simulink model "SWC_VES_type"  (R2021b)
settings: Solver=FixedStepDiscrete  StartTime=0.0  StopTime=10.0  FixedStep=0.001  RelTol=1e-3
undefined symbols (not defined in the file or in its folder): R_HALINCDD_CSOP_IPCF_Handler
libraries: simulink x78
(part 1 of 2)
settings Model: DataDictionary=APPTypes.sldd  Creator=FVT23010  LastModifiedBy=FVT23033
settings DataIOCC: SaveFormat=StructureWithTime
settings OptimizationCC: DefaultParameterBehavior=Inlined  EnhancedBackFolding=on  PassReuseOutputArgsAs=Individual arguments  ZeroExternalMemoryAtStartup=off  ZeroInternalMemoryAtStartup=off  OptimizeBlockOrder=speed  DifferentSizesBufferReuse=on  OptimizationCustomize=off  EfficientTunableParamExpr=on
settings DebuggingCC: ParameterTunabilityLossMsg=error
settings HardwareCC: ProdBitPerPointer=32  ProdBitPerSizeT=32  ProdBitPerPtrDiffT=32  ProdLargestAtomicInteger=Long  ProdLargestAtomicFloat=Double  ProdWordSize=32  ProdLongLongMode=on  ProdHWDeviceType=ARM Compatible->ARM Cortex-M
settings ModelReferenceCC: ModelReferenceNumInstancesAllowed=Single
settings SFSimCC: MATLABDynamicMemAlloc=off
settings RTWCC: Description=AUTOSAR  SystemTargetFile=autosar.tlc  GenCodeOnly=on  TemplateMakefile=ert_default_tmf  PortableWordSizes=on
settings CodeAppCC: ForceParamTrailComments=on  IgnoreCustomStorageClasses=off  OperatorAnnotations=on  SimulinkDataObjDesc=on  SFDataObjDesc=on  InsertBlockDesc=on
settings STFCustomTargetCC: TargetLangStandard=C99 (ISO)  UtilityFuncGeneration=Shared location  MultiwordLength=256  ParMdlRefBuildCompliant=on  CompOptLevelCompliant=on  IncludeMdlTerminateFcn=off  CombineOutputUpdateFcns=on  SuppressErrorStatus=on  ERTCustomFileBanners=on  SupportNonFinite=off  SupportComplex=off  SupportContinuousTime=off  SupportNonInlinedSFcns=off  RemoveResetFunc=on  MATLABClassNameForMDSCustomization=Simulink.SoftwareTarget.ERTCustomization  AutosarCompliant=on  GRTInterface=off  UseToolchainInfoCompliant=on  GenerateSharedConstants=off  LookupTableObjectStructAxisOrder=2,1,3,4,...  LUTObjectStructOrderEvenSpacing=Size,Table,Breakpoints  SystemTargetFile=autosar.tlc
settings ERTTargetCC: TargetLangStandard=C99 (ISO)  UtilityFuncGeneration=Shared location  ConcurrentExecutionCompliant=off  IncludeMdlTerminateFcn=off  SuppressErrorStatus=on  SupportNonFinite=off  SupportComplex=off  ModelStepFunctionPrototypeControlCompliant=off  CPPClassGenCompliant=off  AutosarCompliant=on  GenerateSharedConstants=off  LookupTableObjectStructAxisOrder=2,1,3,4,...  LUTObjectStructOrderEvenSpacing=Size,Table,Breakpoints  GenerateASAP2=on  InlinedParameterPlacement=NonHierarchical  ERTCustomFileTemplate=example_file_process.tlc  ConvertIfToSwitch=off  SuppressUnreachableDefaultCases=off  BooleanTrueId=true_MatlabRTW  BooleanFalseId=false_MatlabRTW

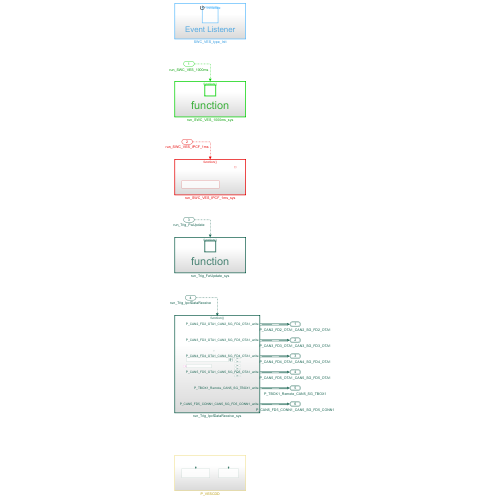
[thumbnail: Simulink's stored preview of the top-level diagram]
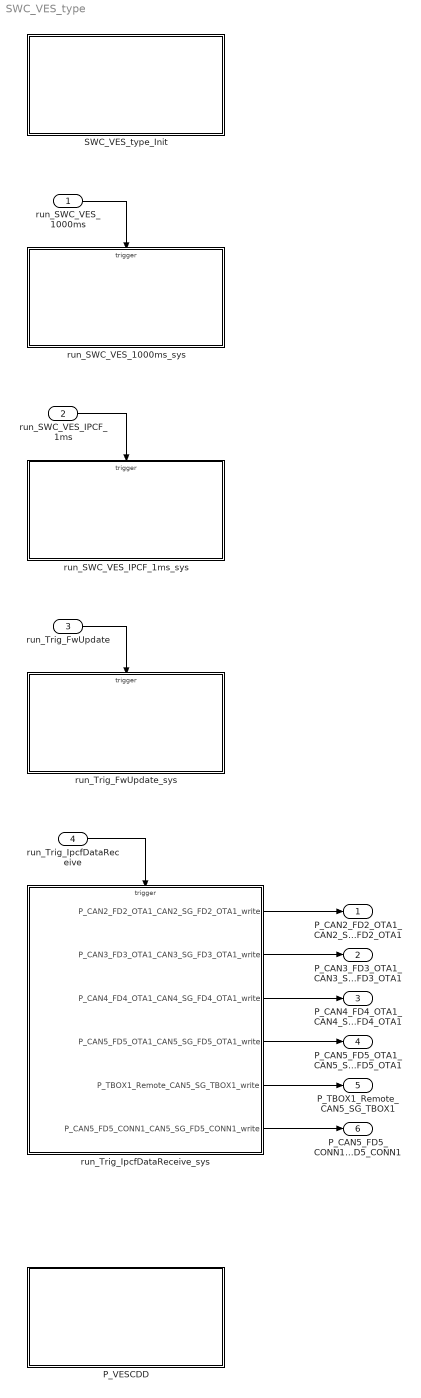
== system SWC_VES_type ==
  run_SWC_VES_1000ms : Inport  SampleTime=1  OutputFunctionCall=on
  run_SWC_VES_IPCF_1ms : Inport  Port=2  SampleTime=0.001  OutputFunctionCall=on
  run_Trig_FwUpdate : Inport  Port=3  OutputFunctionCall=on
  run_Trig_IpcfDataReceive : Inport  Port=4  OutputFunctionCall=on
  P_VESCDD : Subsystem
  SWC_VES_type_Init : Subsystem
  run_SWC_VES_1000ms_sys : Subsystem
  run_SWC_VES_IPCF_1ms_sys : Subsystem
  run_Trig_FwUpdate_sys : Subsystem
  run_Trig_IpcfDataReceive_sys : Subsystem
  P_CAN2_FD2_OTA1_CAN2_SG_FD2_OTA1 : Outport  OutDataTypeStr=Bus: DT_CAN2_SG_FD2_OTA1  PortDimensions=1  BusOutputAsStruct=on
  P_CAN3_FD3_OTA1_CAN3_SG_FD3_OTA1 : Outport  Port=2  OutDataTypeStr=Bus: DT_CAN3_SG_FD3_OTA1  PortDimensions=1  BusOutputAsStruct=on
  P_CAN4_FD4_OTA1_CAN4_SG_FD4_OTA1 : Outport  Port=3  OutDataTypeStr=Bus: DT_CAN4_SG_FD4_OTA1  PortDimensions=1  BusOutputAsStruct=on
  P_CAN5_FD5_OTA1_CAN5_SG_FD5_OTA1 : Outport  Port=4  OutDataTypeStr=Bus: DT_CAN5_SG_FD5_OTA1  PortDimensions=1  BusOutputAsStruct=on
  P_TBOX1_Remote_CAN5_SG_TBOX1 : Outport  Port=5  OutDataTypeStr=Bus: DT_CAN5_SG_TBOX1  PortDimensions=1  BusOutputAsStruct=on
  P_CAN5_FD5_CONN1_CAN5_SG_FD5_CONN1 : Outport  Port=6  OutDataTypeStr=Bus: DT_CAN5_SG_FD5_CONN1  PortDimensions=1  BusOutputAsStruct=on
  wires:
  run_Trig_IpcfDataReceive_sys/1(P_CAN2_FD2_OTA1_CAN2_SG_FD2_OTA1_write) -> P_CAN2_FD2_OTA1_CAN2_SG_FD2_OTA1/1
  run_Trig_IpcfDataReceive_sys/2(P_CAN3_FD3_OTA1_CAN3_SG_FD3_OTA1_write) -> P_CAN3_FD3_OTA1_CAN3_SG_FD3_OTA1/1
  run_Trig_IpcfDataReceive_sys/3(P_CAN4_FD4_OTA1_CAN4_SG_FD4_OTA1_write) -> P_CAN4_FD4_OTA1_CAN4_SG_FD4_OTA1/1
  run_Trig_IpcfDataReceive_sys/4(P_CAN5_FD5_OTA1_CAN5_SG_FD5_OTA1_write) -> P_CAN5_FD5_OTA1_CAN5_SG_FD5_OTA1/1
  run_Trig_IpcfDataReceive_sys/5(P_TBOX1_Remote_CAN5_SG_TBOX1_write) -> P_TBOX1_Remote_CAN5_SG_TBOX1/1
  run_Trig_IpcfDataReceive_sys/6(P_CAN5_FD5_CONN1_CAN5_SG_FD5_CONN1_write) -> P_CAN5_FD5_CONN1_CAN5_SG_FD5_CONN1/1
  run_SWC_VES_1000ms/1 -> run_SWC_VES_1000ms_sys/Trigger
  run_SWC_VES_IPCF_1ms/1 -> run_SWC_VES_IPCF_1ms_sys/Trigger
  run_Trig_FwUpdate/1 -> run_Trig_FwUpdate_sys/Trigger
  run_Trig_IpcfDataReceive/1 -> run_Trig_IpcfDataReceive_sys/Trigger

== system SWC_VES_type/P_VESCDD ==
  run_VESCDD_sys : Subsystem

== system SWC_VES_type/SWC_VES_type_Init ==
  Event Listener : EventListener  EventName=reset

== system SWC_VES_type/run_SWC_VES_1000ms_sys ==
  function : TriggerPort  TriggerType=function-call  VariantControl=(inherit)  SampleTimeType=periodic  SampleTime=-1

== system SWC_VES_type/run_SWC_VES_IPCF_1ms_sys ==
  function : TriggerPort  TriggerType=function-call  VariantControl=(inherit)  SampleTimeType=periodic  SampleTime=-1
  R_HALINCDD_CSOP_IPCF_Handler : FunctionCaller  FunctionPrototype=R_HALINCDD_CSOP_IPCF_Handler()

== system SWC_VES_type/run_Trig_FwUpdate_sys ==
  function : TriggerPort  TriggerType=function-call  VariantControl=(inherit)

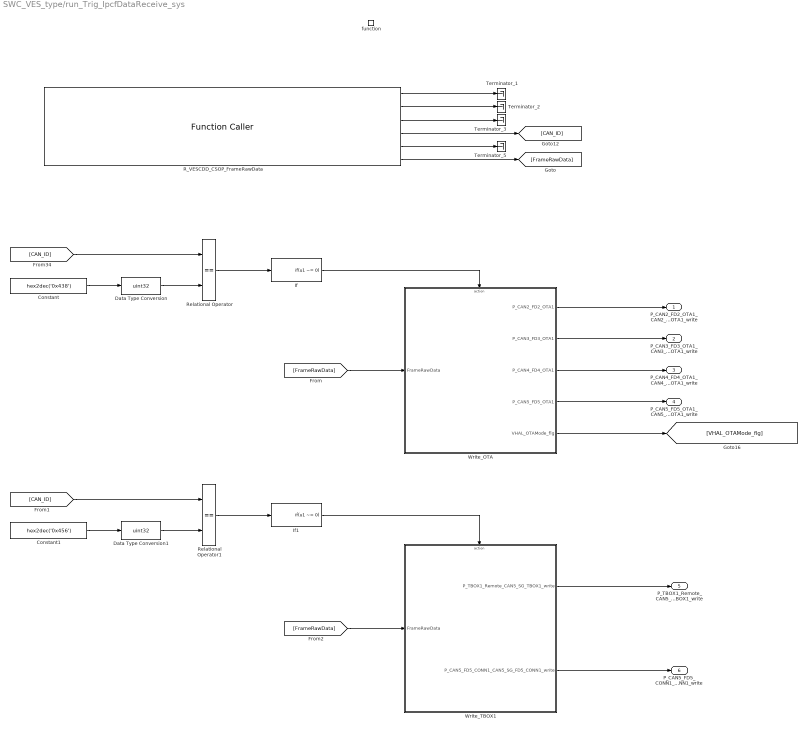
== system SWC_VES_type/run_Trig_IpcfDataReceive_sys ==
  function : TriggerPort  TriggerType=function-call  VariantControl=(inherit)
  Constant : Constant  Value=hex2dec('0x438')
  Constant1 : Constant  Value=hex2dec('0x456')
  Data Type Conversion : DataTypeConversion  OutDataTypeStr=uint32
  Data Type Conversion1 : DataTypeConversion  OutDataTypeStr=uint32
  If : If  IfExpression=u1 ~= 0  ShowElse=off
  If1 : If  IfExpression=u1 ~= 0  ShowElse=off
  R_VESCDD_CSOP_FrameRawData : FunctionCaller  FunctionPrototype=[channel,fd,ext,id,dlc,FrameRawData] = R_VESCDD_CSOP_FrameRawData()  OutputArgumentSpecifications=uint8(1), uint8(1), uint8(1), uint32(1), uint8(1), uint8([1;1;1;1;1;1;1;1;1;1;1;1;1;1;1;1;1;1;1;1;1;1;1;1;1;1;1;1;1;1;1;1;1;1;1;1;1;1;1;1;1;1;1;1;1;1;1;1;1;1;1;1;1;1;1;1;1;1;1;1;1;1;1;1])
  Relational Operator : RelationalOperator  Operator===  OutDataTypeStr=boolean  RndMeth=Simplest
  Relational Operator1 : RelationalOperator  Operator===  OutDataTypeStr=boolean  RndMeth=Simplest
  Terminator_{1..3,5} (4 alike) : Terminator
  Write_OTA : Subsystem  TreatAsAtomicUnit=on
  Write_TBOX1 : Subsystem  TreatAsAtomicUnit=on
  P_CAN2_FD2_OTA1_CAN2_SG_FD2_OTA1_write : Outport
  P_CAN3_FD3_OTA1_CAN3_SG_FD3_OTA1_write : Outport  Port=2
  P_CAN4_FD4_OTA1_CAN4_SG_FD4_OTA1_write : Outport  Port=3
  P_CAN5_FD5_OTA1_CAN5_SG_FD5_OTA1_write : Outport  Port=4
  P_TBOX1_Remote_CAN5_SG_TBOX1_write : Outport  Port=5
  P_CAN5_FD5_CONN1_CAN5_SG_FD5_CONN1_write : Outport  Port=6
  wires:
  R_VESCDD_CSOP_FrameRawData/4 -> [CAN_ID]
  R_VESCDD_CSOP_FrameRawData/5 -> Terminator_5/1
  R_VESCDD_CSOP_FrameRawData/1 -> Terminator_1/1
  R_VESCDD_CSOP_FrameRawData/6 -> [FrameRawData]
  R_VESCDD_CSOP_FrameRawData/3 -> Terminator_3/1
  R_VESCDD_CSOP_FrameRawData/2 -> Terminator_2/1
  [CAN_ID] -> Relational Operator/1
  [FrameRawData] -> Write_OTA/1(FrameRawData)
  Constant/1 -> Data Type Conversion/1
  Relational Operator/1 -> If/1
  If/1 -> Write_OTA/Action
  Data Type Conversion/1 -> Relational Operator/2
  Relational Operator1/1 -> If1/1
  [FrameRawData] -> Write_TBOX1/1(FrameRawData)
  Constant1/1 -> Data Type Conversion1/1
  If1/1 -> Write_TBOX1/Action
  [CAN_ID] -> Relational Operator1/1
  Data Type Conversion1/1 -> Relational Operator1/2
  Write_OTA/1(P_CAN2_FD2_OTA1) -> P_CAN2_FD2_OTA1_CAN2_SG_FD2_OTA1_write/1
  Write_OTA/2(P_CAN3_FD3_OTA1) -> P_CAN3_FD3_OTA1_CAN3_SG_FD3_OTA1_write/1
  Write_OTA/3(P_CAN4_FD4_OTA1) -> P_CAN4_FD4_OTA1_CAN4_SG_FD4_OTA1_write/1
  Write_OTA/4(P_CAN5_FD5_OTA1) -> P_CAN5_FD5_OTA1_CAN5_SG_FD5_OTA1_write/1
  Write_OTA/5(VHAL_OTAMode_flg) -> [VHAL_OTAMode_flg]
  Write_TBOX1/2(P_CAN5_FD5_CONN1_CAN5_SG_FD5_CONN1_write) -> P_CAN5_FD5_CONN1_CAN5_SG_FD5_CONN1_write/1
  Write_TBOX1/1(P_TBOX1_Remote_CAN5_SG_TBOX1_write) -> P_TBOX1_Remote_CAN5_SG_TBOX1_write/1

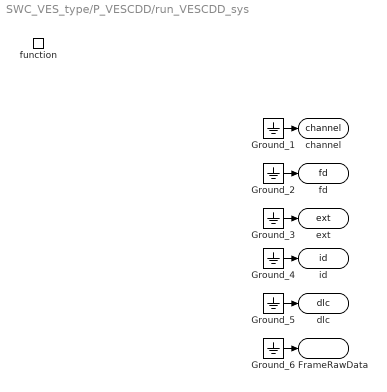
== system SWC_VES_type/P_VESCDD/run_VESCDD_sys ==
  function : TriggerPort  TriggerType=function-call  IsSimulinkFunction=on  FunctionName=run_VESCDD  VariantControl=(inherit)
  Ground_{1..6} (6 alike) : Ground
  channel : ArgOut  OutDataTypeStr=uint8  ArgumentName=channel
  fd : ArgOut  Port=2  OutDataTypeStr=uint8  ArgumentName=fd
  ext : ArgOut  Port=3  OutDataTypeStr=uint8  ArgumentName=ext
  id : ArgOut  Port=4  OutDataTypeStr=uint32  ArgumentName=id
  dlc : ArgOut  Port=5  OutDataTypeStr=uint8  ArgumentName=dlc
  FrameRawData : ArgOut  Port=6  OutDataTypeStr=uint8  PortDimensions=64  ArgumentName=FrameRawData
  wires:
  Ground_1/1 -> channel/1
  Ground_2/1 -> fd/1
  Ground_3/1 -> ext/1
  Ground_4/1 -> id/1
  Ground_5/1 -> dlc/1
  Ground_6/1 -> FrameRawData/1

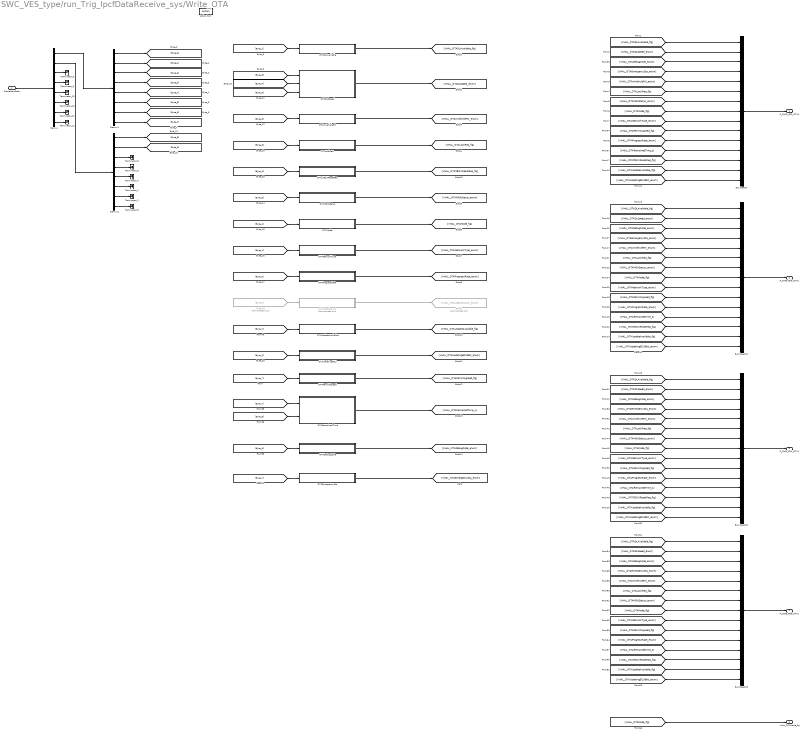
== system SWC_VES_type/run_Trig_IpcfDataReceive_sys/Write_OTA ==
  FrameRawData : Inport
  Action Port : ActionPort  ActionPortLabel=if(u1 ~= 0)
  Bus Creator : BusCreator  Inputs=15  OutDataTypeStr=Bus: DT_CAN2_SG_FD2_OTA1  NonVirtualBus=on
      settings: InheritFromInputs=off
  Bus Creator1 : BusCreator  Inputs=15  OutDataTypeStr=Bus: DT_CAN3_SG_FD3_OTA1  NonVirtualBus=on
      settings: InheritFromInputs=off
  Bus Creator2 : BusCreator  Inputs=15  OutDataTypeStr=Bus: DT_CAN4_SG_FD4_OTA1  NonVirtualBus=on
      settings: InheritFromInputs=off
  Bus Creator3 : BusCreator  Inputs=15  OutDataTypeStr=Bus: DT_CAN5_SG_FD5_OTA1  NonVirtualBus=on
      settings: InheritFromInputs=off
  Byte_18 : From  Commented=on  GotoTag=Byte_6
  Demux : Demux  Outputs=8
  Demux1 : Demux  Outputs=8
  Demux2 : Demux  Outputs=8
  Goto9 : Goto  Commented=on  GotoTag=VHAL_OTAUpBackcount_enum
  OTADLAvailable : Subsystem
  OTADLSpeed : Subsystem
  OTADebugCode : Subsystem
  OTAEmergencySta : Subsystem
  OTAInVehicleFW : Subsystem
  OTALockReq : Subsystem
  OTAMDAStatus : Subsystem
  OTAMode : Subsystem
  OTANetworkType : Subsystem
  OTAPermitAgreed : Subsystem
  OTAProgressRate : Subsystem
  OTARemainedTime : Subsystem
  OTAUpBackcount : Subsystem  Commented=on
  OTAUpdateAvailable : Subsystem
  OTAUpdatingECU : Subsystem
  OTA_TBOXResetReq : Subsystem
  Terminator_{1..6,8..13} (12 alike) : Terminator
  P_CAN2_FD2_OTA1 : Outport
  P_CAN3_FD3_OTA1 : Outport  Port=2
  P_CAN4_FD4_OTA1 : Outport  Port=3
  P_CAN5_FD5_OTA1 : Outport  Port=4
  VHAL_OTAMode_flg : Outport  Port=5
  wires:
  [Byte_2] -> OTAUpdatingECU/1(Byte_2)
  Demux1/7 -> [Byte_6]  "Raw_Byte6"
  Demux1/4 -> [Byte_3]  "Raw_Byte3"
  Demux1/6 -> [Byte_5]  "Raw_Byte5"
  [Byte_5] -> OTADLSpeed/3(Byte_5)
  Demux/1 -> Demux1/1
  [Byte_7] -> OTAUpdateAvailable/1(Byte_7)
  Demux/4 -> Terminator_9/1
  [Byte_3] -> OTALockReq/1(Byte_3)
  [Byte_3] -> OTADLSpeed/1(Byte_3)
  Demux/5 -> Terminator_13/1
  [Byte_4] -> OTADLSpeed/2(Byte_4)
  Byte_18/1 -> OTAUpBackcount/1(Byte_6)
  Demux1/8 -> [Byte_7]  "Raw_Byte7"
  Demux1/3 -> [Byte_2]  "Raw_Byte2"
  Demux1/2 -> [Byte_1]  "Raw_Byte1"
  Demux1/5 -> [Byte_4]  "Raw_Byte4"
  Demux1/1 -> [Byte_0]  "Raw_Byte0"
  [Byte_1] -> OTANetworkType/1(Byte_1)
  Demux/7 -> Terminator_11/1
  FrameRawData/1 -> Demux/1
  [Byte_6] -> OTAMDAStatus/1(Byte_1)
  Demux/3 -> Terminator_8/1
  [Byte_1] -> OTAMode/1(Byte_1)
  [Byte_0] -> OTAProgressRate/1(Byte_0)
  [Byte_3] -> OTAInVehicleFW/1(Byte_3)
  [Byte_1] -> OTADLAvailable/1(Byte_1)
  Demux/8 -> Terminator_12/1
  Demux/6 -> Terminator_10/1
  OTAUpdateAvailable/1(VHAL_OTAUpdateAvailable_flg) -> [VHAL_OTAUpdateAvailable_flg]
  OTAMode/1(VHAL_OTAMode_flg) -> [VHAL_OTAMode_flg]
  OTAInVehicleFW/1(VHAL_OTAInVehicleFW_enum) -> [VHAL_OTAInVehicleFW_enum]
  OTADLAvailable/1(VHAL_OTADLAvailable_flg) -> [VHAL_OTADLAvailable_flg]
  OTANetworkType/1(VHAL_OTANetworkType_enum) -> [VHAL_OTANetworkType_enum]
  OTADLSpeed/1(VHAL_OTADLSpeed_enum) -> [VHAL_OTADLSpeed_enum]
  OTAMDAStatus/1(VHAL_OTAMDAStatus_enum) -> [VHAL_OTAMDAStatus_enum]
  OTAUpdatingECU/1(VHAL_OTAUpdatingECU_enum) -> [VHAL_OTAUpdatingECU8bit_enum]
  OTALockReq/1(VHAL_OTALockReq_flg) -> [VHAL_OTALockReq_flg]
  OTAUpBackcount/1(VHAL_OTAUpBackcount_enum) -> Goto9/1
  OTAProgressRate/1(VHAL_OTAProgressRate_enum) -> [VHAL_OTAProgressRate_enum]
  Demux/2 -> Demux2/1
  Demux2/1 -> [Byte_8]  "Raw_Byte8"
  Demux2/2 -> [Byte_9]  "Raw_Byte9"
  Demux2/3 -> Terminator_5/1
  Demux2/5 -> Terminator_4/1
  Demux2/6 -> Terminator_1/1
  Demux2/7 -> Terminator_2/1
  Demux2/8 -> Terminator_3/1
  [Byte_7] -> OTAPermitAgreed/1(Byte_7)
  OTAPermitAgreed/1(VHAL_OTAPermitAgreed_flg) -> [VHAL_OTAPermitAgreed_flg]
  [Byte_8] -> OTARemainedTime/2(Byte_8)
  [Byte_7] -> OTARemainedTime/1(Byte_7)
  OTARemainedTime/1(VHAL_OTARemainedTime_s) -> [VHAL_OTARemainedTime_s]
  [Byte_9] -> OTADebugCode/1(Byte_9)
  OTADebugCode/1(VHAL_OTADebugCode_enum) -> [VHAL_OTADebugCode_enum]
  [VHAL_OTADLAvailable_flg] -> Bus Creator/1
  [VHAL_OTADebugCode_enum] -> Bus Creator/3
  Bus Creator/1 -> P_CAN2_FD2_OTA1/1
  [VHAL_OTADLSpeed_enum] -> Bus Creator/2
  Demux2/4 -> Terminator_6/1  "Raw_Byte11"
  OTA_TBOXResetReq/1(VHAL_OTALockReq_flg) -> [VHAL_OTATBOXResetReq_flg]
  [Byte_3] -> OTA_TBOXResetReq/1(Byte_3)
  [VHAL_OTAEmergencySta_enum] -> Bus Creator/4
  [VHAL_OTAInVehicleFW_enum] -> Bus Creator/5
  [VHAL_OTALockReq_flg] -> Bus Creator/6
  [VHAL_OTAMDAStatus_enum] -> Bus Creator/7
  [VHAL_OTAMode_flg] -> Bus Creator/8
  [VHAL_OTANetworkType_enum] -> Bus Creator/9
  [VHAL_OTAPermitAgreed_flg] -> Bus Creator/10
  [VHAL_OTAProgressRate_enum] -> Bus Creator/11
  [VHAL_OTARemainedTime_s] -> Bus Creator/12
  [VHAL_OTATBOXResetReq_flg] -> Bus Creator/13
  [VHAL_OTAUpdateAvailable_flg] -> Bus Creator/14
  [VHAL_OTAUpdatingECU8bit_enum] -> Bus Creator/15
  OTAEmergencySta/1(VHAL_OTAEmergencySta_enum) -> [VHAL_OTAEmergencySta_enum]
  [Byte_7] -> OTAEmergencySta/1(Byte_7)
  [VHAL_OTAUpdatingECU8bit_enum] -> Bus Creator1/15
  [VHAL_OTAUpdateAvailable_flg] -> Bus Creator1/14
  [VHAL_OTATBOXResetReq_flg] -> Bus Creator1/13
  [VHAL_OTARemainedTime_s] -> Bus Creator1/12
  [VHAL_OTAProgressRate_enum] -> Bus Creator1/11
  [VHAL_OTAPermitAgreed_flg] -> Bus Creator1/10
  [VHAL_OTANetworkType_enum] -> Bus Creator1/9
  [VHAL_OTAMode_flg] -> Bus Creator1/8
  [VHAL_OTAMDAStatus_enum] -> Bus Creator1/7
  [VHAL_OTALockReq_flg] -> Bus Creator1/6
  [VHAL_OTAInVehicleFW_enum] -> Bus Creator1/5
  [VHAL_OTAEmergencySta_enum] -> Bus Creator1/4
  [VHAL_OTADLSpeed_enum] -> Bus Creator1/2
  Bus Creator1/1 -> P_CAN3_FD3_OTA1/1
  [VHAL_OTADebugCode_enum] -> Bus Creator1/3
  [VHAL_OTADLAvailable_flg] -> Bus Creator1/1
  [VHAL_OTADLAvailable_flg] -> Bus Creator2/1
  [VHAL_OTADebugCode_enum] -> Bus Creator2/3
  Bus Creator2/1 -> P_CAN4_FD4_OTA1/1
  [VHAL_OTADLSpeed_enum] -> Bus Creator2/2
  [VHAL_OTAEmergencySta_enum] -> Bus Creator2/4
  [VHAL_OTAInVehicleFW_enum] -> Bus Creator2/5
  [VHAL_OTALockReq_flg] -> Bus Creator2/6
  [VHAL_OTAMDAStatus_enum] -> Bus Creator2/7
  [VHAL_OTAMode_flg] -> Bus Creator2/8
  [VHAL_OTANetworkType_enum] -> Bus Creator2/9
  [VHAL_OTAPermitAgreed_flg] -> Bus Creator2/10
  [VHAL_OTAProgressRate_enum] -> Bus Creator2/11
  [VHAL_OTARemainedTime_s] -> Bus Creator2/12
  [VHAL_OTATBOXResetReq_flg] -> Bus Creator2/13
  [VHAL_OTAUpdateAvailable_flg] -> Bus Creator2/14
  [VHAL_OTAUpdatingECU8bit_enum] -> Bus Creator2/15
  [VHAL_OTAUpdatingECU8bit_enum] -> Bus Creator3/15
  [VHAL_OTAUpdateAvailable_flg] -> Bus Creator3/14
  [VHAL_OTATBOXResetReq_flg] -> Bus Creator3/13
  [VHAL_OTARemainedTime_s] -> Bus Creator3/12
  [VHAL_OTAProgressRate_enum] -> Bus Creator3/11
  [VHAL_OTAPermitAgreed_flg] -> Bus Creator3/10
  [VHAL_OTANetworkType_enum] -> Bus Creator3/9
  [VHAL_OTAMode_flg] -> Bus Creator3/8
  [VHAL_OTAMDAStatus_enum] -> Bus Creator3/7
  [VHAL_OTALockReq_flg] -> Bus Creator3/6
  [VHAL_OTAInVehicleFW_enum] -> Bus Creator3/5
  [VHAL_OTAEmergencySta_enum] -> Bus Creator3/4
  [VHAL_OTADLSpeed_enum] -> Bus Creator3/2
  Bus Creator3/1 -> P_CAN5_FD5_OTA1/1
  [VHAL_OTADebugCode_enum] -> Bus Creator3/3
  [VHAL_OTADLAvailable_flg] -> Bus Creator3/1
  [VHAL_OTAMode_flg] -> VHAL_OTAMode_flg/1

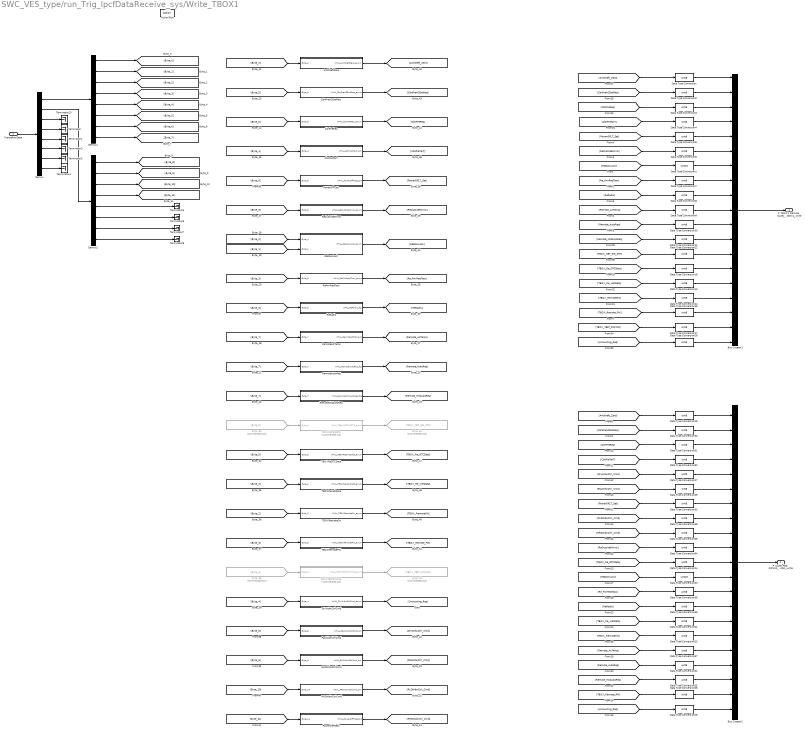
== system SWC_VES_type/run_Trig_IpcfDataReceive_sys/Write_TBOX1 ==
  FrameRawData : Inport
  Action Port : ActionPort  ActionPortLabel=if(u1 ~= 0)
  AntitheftZero : Subsystem
  Bus Creator1 : BusCreator  Inputs=19  OutDataTypeStr=Bus: DT_CAN5_SG_TBOX1  NonVirtualBus=on
      settings: InheritFromInputs=off
  Bus Creator2 : BusCreator  Inputs=21  OutDataTypeStr=Bus: DT_CAN5_SG_FD5_CONN1  NonVirtualBus=on
      settings: InheritFromInputs=off
  Byte_33 : From  Commented=on  GotoTag=Byte_6
  Byte_38 : From  Commented=on  GotoTag=Byte_6
  Byte_49 : Goto  Commented=on  GotoTag=TBOX_TEST_STATUS
  Byte_50 : Goto  Commented=on  GotoTag=TBOX_NET_SIG_STR
  CbnPreACEnaReq : Subsystem
  CbnPreReq : Subsystem
  CbnPreTarT : Subsystem
  Data Type Conversion{,2..19,21..39} (38 alike) : DataTypeConversion  OutDataTypeStr=uint8
  Data Type Conversion1 : DataTypeConversion  OutDataTypeStr=uint16
  Data Type Conversion20 : DataTypeConversion  OutDataTypeStr=uint16
  Demux : Demux  Outputs=8
  Demux1 : Demux  Outputs=8
  Demux2 : Demux  Outputs=8
  DrvWdwCtrlCmd : Subsystem
  PasWdwCtrlCmd : Subsystem
  PowerOffTSet : Subsystem
  PowerOffTSet4 : Subsystem
  RLDWdwCtrlCmd : Subsystem
  RRDWdwCtrlCmd : Subsystem
  ReDoorLock : Subsystem
  ReOutsideMirror : Subsystem
  RePwrReqTbox : Subsystem
  ReRadio : Subsystem
  RemoteACTemp : Subsystem
  RemoteAutoReq : Subsystem
  RemoteMidAutoReq : Subsystem
  TBOXNETSIGSTR : Subsystem  Commented=on
  TBOXReDTCData : Subsystem
  TBOXReVehData : Subsystem
  TBOXRemoteOn : Subsystem
  TBOXRemotePW : Subsystem
  TBOXTESTSTATUS : Subsystem  Commented=on
  Terminator{,1..8,13} (10 alike) : Terminator
  P_TBOX1_Remote_CAN5_SG_TBOX1_write : Outport
  P_CAN5_FD5_CONN1_CAN5_SG_FD5_CONN1_write : Outport  Port=2
  wires:
  Demux/6 -> Terminator2/1
  Demux/7 -> Terminator3/1
  Demux/8 -> Terminator4/1
  Demux/4 -> Terminator/1
  Demux/3 -> Terminator13/1
  FrameRawData/1 -> Demux/1
  Demux/5 -> Terminator1/1
  Demux1/1 -> [Byte_0]
  Demux1/2 -> [Byte_1]
  Demux1/3 -> [Byte_2]
  Demux1/4 -> [Byte_3]
  Demux1/5 -> [Byte_4]
  Demux1/6 -> [Byte_5]
  Demux1/7 -> [Byte_6]
  Demux1/8 -> [Byte_7]
  Demux2/1 -> [Byte_8]
  Demux2/2 -> [Byte_9]
  Demux2/3 -> [Byte_10]
  Demux2/4 -> [Byte_11]
  Bus Creator1/1 -> P_TBOX1_Remote_CAN5_SG_TBOX1_write/1
  [Antitheft_Zero] -> Data Type Conversion/1
  [CbnPreACEnaReq] -> Data Type Conversion2/1
  [CbnPreReq] -> Data Type Conversion3/1
  [CbnPreTarT] -> Data Type Conversion4/1
  [PowerOff_T_Set] -> Data Type Conversion5/1
  [ReOutsideMirror] -> Data Type Conversion6/1
  [ReDoorLock] -> Data Type Conversion1/1
  [Remote_MidAutoReq] -> Data Type Conversion11/1
  [TBOX_Re_DTCData] -> Data Type Conversion16/1
  [TBOX_Re_VehData] -> Data Type Conversion13/1
  [TBOX_TEST_STATUS] -> Data Type Conversion17/1
  [Uncounting_Req] -> Data Type Conversion18/1
  [TBOX_RemoteON] -> Data Type Conversion14/1
  Data Type Conversion1/1 -> Bus Creator1/7
  Data Type Conversion/1 -> Bus Creator1/1
  Data Type Conversion2/1 -> Bus Creator1/2
  Data Type Conversion3/1 -> Bus Creator1/3
  Data Type Conversion6/1 -> Bus Creator1/6
  Data Type Conversion4/1 -> Bus Creator1/4
  Data Type Conversion5/1 -> Bus Creator1/5
  Data Type Conversion12/1 -> Bus Creator1/13
  Data Type Conversion10/1 -> Bus Creator1/11
  Data Type Conversion8/1 -> Bus Creator1/9
  Data Type Conversion9/1 -> Bus Creator1/10
  Data Type Conversion7/1 -> Bus Creator1/8
  Data Type Conversion11/1 -> Bus Creator1/12
  Data Type Conversion16/1 -> Bus Creator1/14
  Data Type Conversion14/1 -> Bus Creator1/16
  Data Type Conversion15/1 -> Bus Creator1/17
  Data Type Conversion13/1 -> Bus Creator1/15
  Data Type Conversion18/1 -> Bus Creator1/19
  Data Type Conversion17/1 -> Bus Creator1/18
  Demux2/5 -> Terminator5/1
  Demux2/6 -> Terminator6/1
  Demux2/7 -> Terminator7/1
  Demux2/8 -> Terminator8/1
  Demux/1 -> Demux1/1
  Demux/2 -> Demux2/1
  [Re_PwrReqTbox] -> Data Type Conversion7/1
  [Remote_AcTemp] -> Data Type Conversion9/1
  [Remote_AutoReq] -> Data Type Conversion10/1
  [ReRadio] -> Data Type Conversion8/1
  [TBOX_Remote_PW] -> Data Type Conversion15/1
  TBOXTESTSTATUS/1(VHAL_TBOXTESTSTATUS_enum) -> Byte_49/1
  TBOXRemoteOn/1(VHAL_TBOXRemoteOn_enum) -> [TBOX_RemoteON]
  TBOXRemotePW/1(VHAL_TBOXRemotePW_enum) -> [TBOX_Remote_PW]
  TBOXNETSIGSTR/1(VHAL_TBOXNETSIGSTR_enum) -> Byte_50/1
  TBOXReVehData/1(VHAL_TBOXReVehData_enum) -> [TBOX_Re_VehData]
  [Byte_5] -> ReOutsideMirror/1(Byte_5)
  RemoteAutoReq/1(VHAL_RemoteAutoReq_flg) -> [Remote_AutoReq]
  [Byte_4] -> DrvWdwCtrlCmd/1(Byte_4)
  ReOutsideMirror/1(VHAL_ReOutsideMirror_enum) -> [ReOutsideMirror]
  TBOXReDTCData/1(VHAL_TBOXReDTCData_enum) -> [TBOX_Re_DTCData]
  [Byte_1] -> ReDoorLock/2(Byte_1)
  [Byte_2] -> TBOXReVehData/1(Byte_2)
  [Byte_6] -> ReRadio/1(Byte_6)
  [Byte_3] -> RePwrReqTbox/1(Byte_3)
  Byte_38/1 -> TBOXTESTSTATUS/1(Byte_6)
  [Byte_0] -> ReDoorLock/1(Byte_0)
  ReDoorLock/1(VHAL_ReDoorLock_enum) -> [ReDoorLock]
  RemoteMidAutoReq/1(VHAL_RemoteMidAutoReq_flg) -> [Remote_MidAutoReq]
  [Byte_5] -> CbnPreACEnaReq/1(Byte_5)
  AntitheftZero/1(VHAL_AntitheftZero_enum) -> [Antitheft_Zero]
  [Byte_3] -> TBOXRemotePW/1(Byte_3)
  [Byte_6] -> PowerOffTSet/1(Byte_6)
  [Byte_2] -> AntitheftZero/1(Byte_2)
  [Byte_4] -> CbnPreTarT/1(Byte_4)
  CbnPreACEnaReq/1(VHAL_CbnPreACEnaReq_enum) -> [CbnPreACEnaReq]
  Byte_33/1 -> TBOXNETSIGSTR/1(Byte_6)
  [Byte_5] -> CbnPreReq/1(Byte_5)
  [Byte_2] -> TBOXRemoteOn/1(Byte_2)
  CbnPreReq/1(VHAL_CbnPreReq_enum) -> [CbnPreReq]
  CbnPreTarT/1(VHAL_CbnPreTarT_cnt) -> [CbnPreTarT]
  [Byte_5] -> TBOXReDTCData/1(Byte_5)
  PowerOffTSet/1(VHAL_PowerOffTSet_cnt) -> [PowerOff_T_Set]
  RePwrReqTbox/1(VHAL_RePwrReqTbox_enum) -> [Re_PwrReqTbox]
  ReRadio/1(VHAL_ReRadio_flg) -> [ReRadio]
  RemoteACTemp/1(VHAL_RemoteACTemp_C) -> [Remote_AcTemp]
  [Remote_AcTemp] -> Data Type Conversion37/1
  [CbnPreACEnaReq] -> Data Type Conversion30/1
  [Remote_AutoReq] -> Data Type Conversion21/1
  [ReRadio] -> Data Type Conversion36/1
  [Re_PwrReqTbox] -> Data Type Conversion35/1
  [TBOX_Remote_PW] -> Data Type Conversion26/1
  [Antitheft_Zero] -> Data Type Conversion19/1
  [ReOutsideMirror] -> Data Type Conversion34/1
  [PowerOff_T_Set] -> Data Type Conversion33/1
  [Uncounting_Req] -> Data Type Conversion28/1
  Bus Creator2/1 -> P_CAN5_FD5_CONN1_CAN5_SG_FD5_CONN1_write/1
  [ReDoorLock] -> Data Type Conversion20/1
  [CbnPreReq] -> Data Type Conversion31/1
  [CbnPreTarT] -> Data Type Conversion32/1
  [TBOX_Re_VehData] -> Data Type Conversion22/1
  [TBOX_RemoteON] -> Data Type Conversion23/1
  [TBOX_Re_DTCData] -> Data Type Conversion24/1
  [Remote_MidAutoReq] -> Data Type Conversion25/1
  [TBOX_NET_SIG_STR] -> Data Type Conversion12/1
  [Byte_7] -> RemoteACTemp/1(Byte_7)
  [Byte_7] -> RemoteAutoReq/1(Byte_7)
  [Byte_7] -> RemoteMidAutoReq/1(Byte_7)
  [Byte_8] -> PasWdwCtrlCmd/1(Byte_8)
  [Byte_9] -> RLDWdwCtrlCmd/1(Byte_9)
  [Byte_10] -> RRDWdwCtrlCmd/1(Byte_10)
  [Byte_11] -> PowerOffTSet4/1(Byte_11)
  DrvWdwCtrlCmd/1(VHAL_DrvWdwCtrlCmd_enum) -> [Uncounting_Req]
  PasWdwCtrlCmd/1(VHAL_PasWdwCtrlCmd_cnt) -> [DrvWdwCtrl_Cmd]
  RLDWdwCtrlCmd/1(VHAL_RLDWdwCtrlCmd_cnt) -> [PasWdwCtrl_Cmd]
  RRDWdwCtrlCmd/1(VHAL_RRDWdwCtrlCmd_cnt) -> [RLDWdwCtrl_Cmd]
  PowerOffTSet4/1(VHAL_PowerOffTSet_cnt) -> [RRDWdwCtrl_Cmd]
  [DrvWdwCtrl_Cmd] -> Data Type Conversion27/1
  [PasWdwCtrl_Cmd] -> Data Type Conversion29/1
  [RLDWdwCtrl_Cmd] -> Data Type Conversion38/1
  [RRDWdwCtrl_Cmd] -> Data Type Conversion39/1
  Data Type Conversion30/1 -> Bus Creator2/2
  Data Type Conversion32/1 -> Bus Creator2/4
  Data Type Conversion19/1 -> Bus Creator2/1
  Data Type Conversion31/1 -> Bus Creator2/3
  Data Type Conversion29/1 -> Bus Creator2/6
  Data Type Conversion27/1 -> Bus Creator2/5
  Data Type Conversion38/1 -> Bus Creator2/8
  Data Type Conversion33/1 -> Bus Creator2/7
  Data Type Conversion39/1 -> Bus Creator2/9
  Data Type Conversion34/1 -> Bus Creator2/10
  Data Type Conversion24/1 -> Bus Creator2/11
  Data Type Conversion20/1 -> Bus Creator2/12
  Data Type Conversion35/1 -> Bus Creator2/13
  Data Type Conversion36/1 -> Bus Creator2/14
  Data Type Conversion22/1 -> Bus Creator2/15
  Data Type Conversion23/1 -> Bus Creator2/16
  Data Type Conversion37/1 -> Bus Creator2/17
  Data Type Conversion21/1 -> Bus Creator2/18
  Data Type Conversion25/1 -> Bus Creator2/19
  Data Type Conversion26/1 -> Bus Creator2/20
  Data Type Conversion28/1 -> Bus Creator2/21

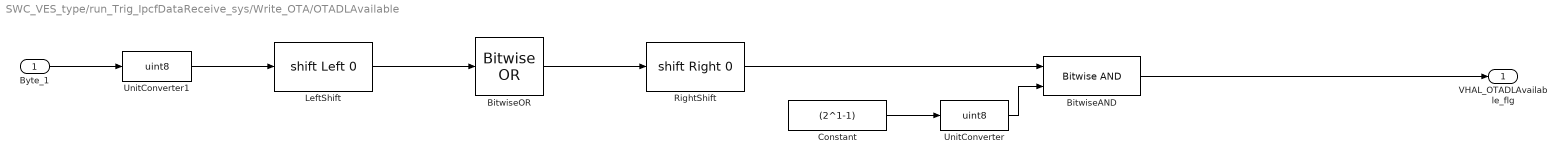
== system SWC_VES_type/run_Trig_IpcfDataReceive_sys/Write_OTA/OTADLAvailable ==
  Byte_1 : Inport
  BitwiseAND : simulink/Logic and Bit Operations/Bitwise Operator  logicop=AND  UseBitMask=off  NumInputPorts=2  BitMask=bin2dec('11011001')  BitMaskRealWorld=Stored Integer
  BitwiseOR : simulink/Logic and Bit Operations/Bitwise Operator  logicop=OR  UseBitMask=off  BitMask=bin2dec('11011001')  BitMaskRealWorld=Stored Integer
  Constant : Constant  Value=(2^1-1)
  LeftShift : ArithShift  BitShiftDirection=Left
  RightShift : ArithShift  BitShiftDirection=Right
  UnitConverter : DataTypeConversion  OutDataTypeStr=uint8
  UnitConverter1 : DataTypeConversion  OutDataTypeStr=uint8
  VHAL_OTADLAvailable_flg : Outport
  wires:
  BitwiseOR/1 -> RightShift/1
  RightShift/1 -> BitwiseAND/1
  UnitConverter/1 -> BitwiseAND/2
  Constant/1 -> UnitConverter/1
  BitwiseAND/1 -> VHAL_OTADLAvailable_flg/1
  LeftShift/1 -> BitwiseOR/1
  UnitConverter1/1 -> LeftShift/1
  Byte_1/1 -> UnitConverter1/1

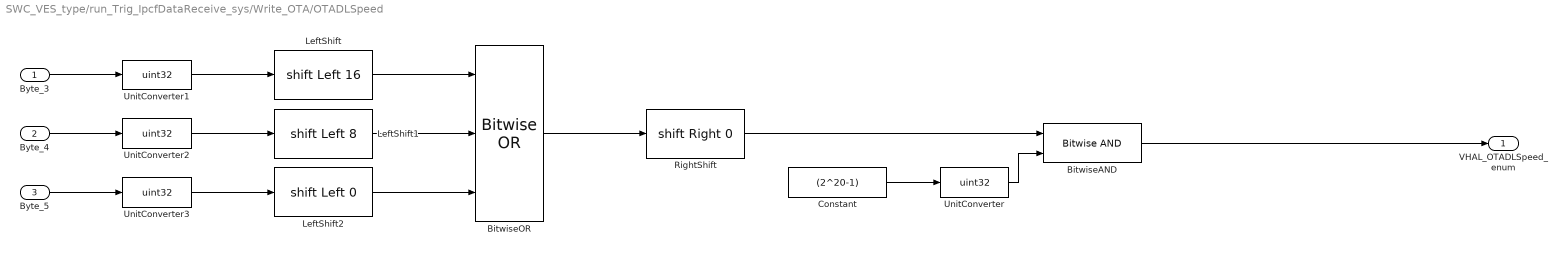
== system SWC_VES_type/run_Trig_IpcfDataReceive_sys/Write_OTA/OTADLSpeed ==
  Byte_3 : Inport
  Byte_4 : Inport  Port=2
  Byte_5 : Inport  Port=3
  BitwiseAND : simulink/Logic and Bit Operations/Bitwise Operator  logicop=AND  UseBitMask=off  NumInputPorts=2  BitMask=bin2dec('11011001')  BitMaskRealWorld=Stored Integer
  BitwiseOR : simulink/Logic and Bit Operations/Bitwise Operator  logicop=OR  UseBitMask=off  NumInputPorts=3  BitMask=bin2dec('11011001')  BitMaskRealWorld=Stored Integer
  Constant : Constant  Value=(2^20-1)
  LeftShift : ArithShift  BitShiftNumber=16  BitShiftDirection=Left
  LeftShift1 : ArithShift  BitShiftNumber=8  BitShiftDirection=Left
  LeftShift2 : ArithShift  BitShiftDirection=Left
  RightShift : ArithShift  BitShiftDirection=Right
  UnitConverter{,1..3} (4 alike) : DataTypeConversion  OutDataTypeStr=uint32
  VHAL_OTADLSpeed_enum : Outport
  wires:
  BitwiseOR/1 -> RightShift/1
  RightShift/1 -> BitwiseAND/1
  UnitConverter/1 -> BitwiseAND/2
  Constant/1 -> UnitConverter/1
  BitwiseAND/1 -> VHAL_OTADLSpeed_enum/1
  LeftShift/1 -> BitwiseOR/1
  UnitConverter1/1 -> LeftShift/1
  Byte_3/1 -> UnitConverter1/1
  LeftShift1/1 -> BitwiseOR/2
  UnitConverter2/1 -> LeftShift1/1
  Byte_4/1 -> UnitConverter2/1
  LeftShift2/1 -> BitwiseOR/3
  UnitConverter3/1 -> LeftShift2/1
  Byte_5/1 -> UnitConverter3/1

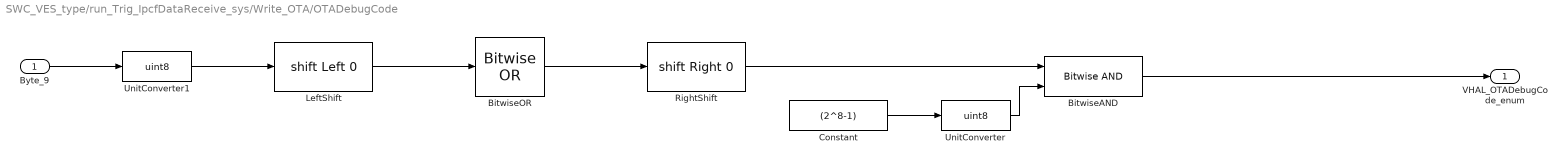
== system SWC_VES_type/run_Trig_IpcfDataReceive_sys/Write_OTA/OTADebugCode ==
  Byte_9 : Inport
  BitwiseAND : simulink/Logic and Bit Operations/Bitwise Operator  logicop=AND  UseBitMask=off  NumInputPorts=2  BitMask=bin2dec('11011001')  BitMaskRealWorld=Stored Integer
  BitwiseOR : simulink/Logic and Bit Operations/Bitwise Operator  logicop=OR  UseBitMask=off  BitMask=bin2dec('11011001')  BitMaskRealWorld=Stored Integer
  Constant : Constant  Value=(2^8-1)
  LeftShift : ArithShift  BitShiftDirection=Left
  RightShift : ArithShift  BitShiftDirection=Right
  UnitConverter : DataTypeConversion  OutDataTypeStr=uint8
  UnitConverter1 : DataTypeConversion  OutDataTypeStr=uint8
  VHAL_OTADebugCode_enum : Outport
  wires:
  BitwiseOR/1 -> RightShift/1
  RightShift/1 -> BitwiseAND/1
  UnitConverter/1 -> BitwiseAND/2
  Constant/1 -> UnitConverter/1
  BitwiseAND/1 -> VHAL_OTADebugCode_enum/1
  LeftShift/1 -> BitwiseOR/1
  UnitConverter1/1 -> LeftShift/1
  Byte_9/1 -> UnitConverter1/1

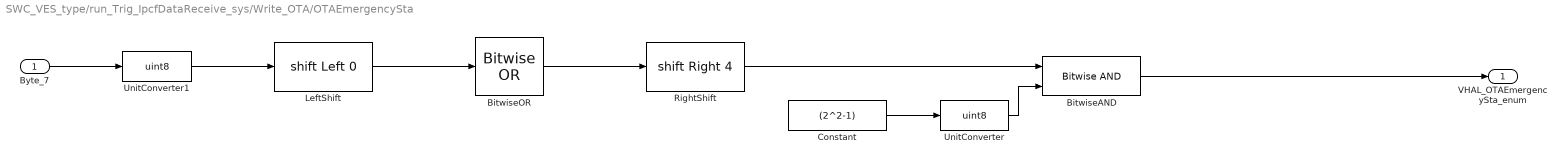
== system SWC_VES_type/run_Trig_IpcfDataReceive_sys/Write_OTA/OTAEmergencySta ==
  Byte_7 : Inport
  BitwiseAND : simulink/Logic and Bit Operations/Bitwise Operator  logicop=AND  UseBitMask=off  NumInputPorts=2  BitMask=bin2dec('11011001')  BitMaskRealWorld=Stored Integer
  BitwiseOR : simulink/Logic and Bit Operations/Bitwise Operator  logicop=OR  UseBitMask=off  BitMask=bin2dec('11011001')  BitMaskRealWorld=Stored Integer
  Constant : Constant  Value=(2^2-1)
  LeftShift : ArithShift  BitShiftDirection=Left
  RightShift : ArithShift  BitShiftNumber=4  BitShiftDirection=Right
  UnitConverter : DataTypeConversion  OutDataTypeStr=uint8
  UnitConverter1 : DataTypeConversion  OutDataTypeStr=uint8
  VHAL_OTAEmergencySta_enum : Outport
  wires:
  Byte_7/1 -> UnitConverter1/1
  UnitConverter1/1 -> LeftShift/1
  LeftShift/1 -> BitwiseOR/1
  BitwiseAND/1 -> VHAL_OTAEmergencySta_enum/1
  Constant/1 -> UnitConverter/1
  UnitConverter/1 -> BitwiseAND/2
  RightShift/1 -> BitwiseAND/1
  BitwiseOR/1 -> RightShift/1

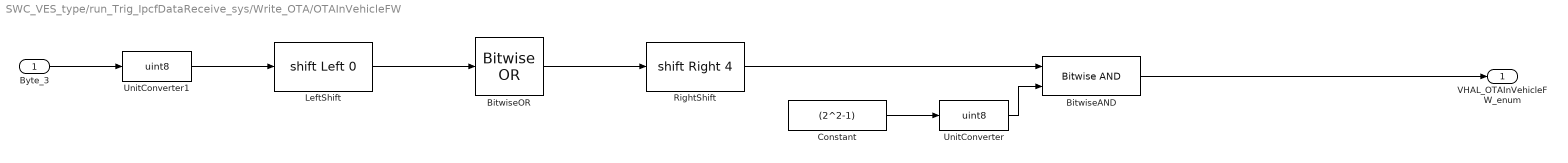
== system SWC_VES_type/run_Trig_IpcfDataReceive_sys/Write_OTA/OTAInVehicleFW ==
  Byte_3 : Inport
  BitwiseAND : simulink/Logic and Bit Operations/Bitwise Operator  logicop=AND  UseBitMask=off  NumInputPorts=2  BitMask=bin2dec('11011001')  BitMaskRealWorld=Stored Integer
  BitwiseOR : simulink/Logic and Bit Operations/Bitwise Operator  logicop=OR  UseBitMask=off  BitMask=bin2dec('11011001')  BitMaskRealWorld=Stored Integer
  Constant : Constant  Value=(2^2-1)
  LeftShift : ArithShift  BitShiftDirection=Left
  RightShift : ArithShift  BitShiftNumber=4  BitShiftDirection=Right
  UnitConverter : DataTypeConversion  OutDataTypeStr=uint8
  UnitConverter1 : DataTypeConversion  OutDataTypeStr=uint8
  VHAL_OTAInVehicleFW_enum : Outport
  wires:
  BitwiseOR/1 -> RightShift/1
  RightShift/1 -> BitwiseAND/1
  UnitConverter/1 -> BitwiseAND/2
  Constant/1 -> UnitConverter/1
  BitwiseAND/1 -> VHAL_OTAInVehicleFW_enum/1
  LeftShift/1 -> BitwiseOR/1
  UnitConverter1/1 -> LeftShift/1
  Byte_3/1 -> UnitConverter1/1

== system SWC_VES_type/run_Trig_IpcfDataReceive_sys/Write_OTA/OTALockReq ==
  Byte_3 : Inport
  BitwiseAND : simulink/Logic and Bit Operations/Bitwise Operator  logicop=AND  UseBitMask=off  NumInputPorts=2  BitMask=bin2dec('11011001')  BitMaskRealWorld=Stored Integer
  BitwiseOR : simulink/Logic and Bit Operations/Bitwise Operator  logicop=OR  UseBitMask=off  BitMask=bin2dec('11011001')  BitMaskRealWorld=Stored Integer
  Constant : Constant  Value=(2^1-1)
  LeftShift : ArithShift  BitShiftDirection=Left
  RightShift : ArithShift  BitShiftNumber=7  BitShiftDirection=Right
  UnitConverter : DataTypeConversion  OutDataTypeStr=uint8
  UnitConverter1 : DataTypeConversion  OutDataTypeStr=uint8
  VHAL_OTALockReq_flg : Outport
  wires:
  BitwiseOR/1 -> RightShift/1
  RightShift/1 -> BitwiseAND/1
  UnitConverter/1 -> BitwiseAND/2
  Constant/1 -> UnitConverter/1
  BitwiseAND/1 -> VHAL_OTALockReq_flg/1
  LeftShift/1 -> BitwiseOR/1
  UnitConverter1/1 -> LeftShift/1
  Byte_3/1 -> UnitConverter1/1

== system SWC_VES_type/run_Trig_IpcfDataReceive_sys/Write_OTA/OTAMDAStatus ==
  Byte_1 : Inport
  BitwiseAND : simulink/Logic and Bit Operations/Bitwise Operator  logicop=AND  UseBitMask=off  NumInputPorts=2  BitMask=bin2dec('11011001')  BitMaskRealWorld=Stored Integer
  BitwiseOR : simulink/Logic and Bit Operations/Bitwise Operator  logicop=OR  UseBitMask=off  BitMask=bin2dec('11011001')  BitMaskRealWorld=Stored Integer
  Constant : Constant  Value=(2^5-1)
  LeftShift : ArithShift  BitShiftDirection=Left
  RightShift : ArithShift  BitShiftDirection=Right
  UnitConverter : DataTypeConversion  OutDataTypeStr=uint8
  UnitConverter1 : DataTypeConversion  OutDataTypeStr=uint8
  VHAL_OTAMDAStatus_enum : Outport
  wires:
  BitwiseOR/1 -> RightShift/1
  RightShift/1 -> BitwiseAND/1
  UnitConverter/1 -> BitwiseAND/2
  Constant/1 -> UnitConverter/1
  BitwiseAND/1 -> VHAL_OTAMDAStatus_enum/1
  LeftShift/1 -> BitwiseOR/1
  UnitConverter1/1 -> LeftShift/1
  Byte_1/1 -> UnitConverter1/1

== system SWC_VES_type/run_Trig_IpcfDataReceive_sys/Write_OTA/OTAMode ==
  Byte_1 : Inport
  BitwiseAND : simulink/Logic and Bit Operations/Bitwise Operator  logicop=AND  UseBitMask=off  NumInputPorts=2  BitMask=bin2dec('11011001')  BitMaskRealWorld=Stored Integer
  BitwiseOR : simulink/Logic and Bit Operations/Bitwise Operator  logicop=OR  UseBitMask=off  BitMask=bin2dec('11011001')  BitMaskRealWorld=Stored Integer
  Constant : Constant  Value=(2^1-1)
  LeftShift : ArithShift  BitShiftDirection=Left
  RightShift : ArithShift  BitShiftNumber=1  BitShiftDirection=Right
  UnitConverter : DataTypeConversion  OutDataTypeStr=uint8
  UnitConverter1 : DataTypeConversion  OutDataTypeStr=uint8
  VHAL_OTAMode_flg : Outport
  wires:
  BitwiseOR/1 -> RightShift/1
  RightShift/1 -> BitwiseAND/1
  UnitConverter/1 -> BitwiseAND/2
  Constant/1 -> UnitConverter/1
  BitwiseAND/1 -> VHAL_OTAMode_flg/1
  LeftShift/1 -> BitwiseOR/1
  UnitConverter1/1 -> LeftShift/1
  Byte_1/1 -> UnitConverter1/1

== system SWC_VES_type/run_Trig_IpcfDataReceive_sys/Write_OTA/OTANetworkType ==
  Byte_1 : Inport
  BitwiseAND : simulink/Logic and Bit Operations/Bitwise Operator  logicop=AND  UseBitMask=off  NumInputPorts=2  BitMask=bin2dec('11011001')  BitMaskRealWorld=Stored Integer
  BitwiseOR : simulink/Logic and Bit Operations/Bitwise Operator  logicop=OR  UseBitMask=off  BitMask=bin2dec('11011001')  BitMaskRealWorld=Stored Integer
  Constant : Constant  Value=(2^2-1)
  LeftShift : ArithShift  BitShiftDirection=Left
  RightShift : ArithShift  BitShiftNumber=2  BitShiftDirection=Right
  UnitConverter : DataTypeConversion  OutDataTypeStr=uint8
  UnitConverter1 : DataTypeConversion  OutDataTypeStr=uint8
  VHAL_OTANetworkType_enum : Outport
  wires:
  BitwiseOR/1 -> RightShift/1
  RightShift/1 -> BitwiseAND/1
  UnitConverter/1 -> BitwiseAND/2
  Constant/1 -> UnitConverter/1
  BitwiseAND/1 -> VHAL_OTANetworkType_enum/1
  LeftShift/1 -> BitwiseOR/1
  UnitConverter1/1 -> LeftShift/1
  Byte_1/1 -> UnitConverter1/1

== system SWC_VES_type/run_Trig_IpcfDataReceive_sys/Write_OTA/OTAPermitAgreed ==
  Byte_7 : Inport
  BitwiseAND : simulink/Logic and Bit Operations/Bitwise Operator  logicop=AND  UseBitMask=off  NumInputPorts=2  BitMask=bin2dec('11011001')  BitMaskRealWorld=Stored Integer
  BitwiseOR : simulink/Logic and Bit Operations/Bitwise Operator  logicop=OR  UseBitMask=off  BitMask=bin2dec('11011001')  BitMaskRealWorld=Stored Integer
  Constant : Constant  Value=(2^1-1)
  LeftShift : ArithShift  BitShiftDirection=Left
  RightShift : ArithShift  BitShiftNumber=7  BitShiftDirection=Right
  UnitConverter : DataTypeConversion  OutDataTypeStr=uint8
  UnitConverter1 : DataTypeConversion  OutDataTypeStr=uint8
  VHAL_OTAPermitAgreed_flg : Outport
  wires:
  Byte_7/1 -> UnitConverter1/1
  UnitConverter1/1 -> LeftShift/1
  LeftShift/1 -> BitwiseOR/1
  BitwiseAND/1 -> VHAL_OTAPermitAgreed_flg/1
  Constant/1 -> UnitConverter/1
  UnitConverter/1 -> BitwiseAND/2
  RightShift/1 -> BitwiseAND/1
  BitwiseOR/1 -> RightShift/1

== system SWC_VES_type/run_Trig_IpcfDataReceive_sys/Write_OTA/OTAProgressRate ==
  Byte_0 : Inport
  BitwiseAND : simulink/Logic and Bit Operations/Bitwise Operator  logicop=AND  UseBitMask=off  NumInputPorts=2  BitMask=bin2dec('11011001')  BitMaskRealWorld=Stored Integer
  BitwiseOR : simulink/Logic and Bit Operations/Bitwise Operator  logicop=OR  UseBitMask=off  BitMask=bin2dec('11011001')  BitMaskRealWorld=Stored Integer
  Constant : Constant  Value=(2^8-1)
  LeftShift : ArithShift  BitShiftDirection=Left
  RightShift : ArithShift  BitShiftDirection=Right
  UnitConverter : DataTypeConversion  OutDataTypeStr=uint8
  UnitConverter1 : DataTypeConversion  OutDataTypeStr=uint8
  VHAL_OTAProgressRate_enum : Outport
  wires:
  BitwiseOR/1 -> RightShift/1
  RightShift/1 -> BitwiseAND/1
  UnitConverter/1 -> BitwiseAND/2
  Constant/1 -> UnitConverter/1
  BitwiseAND/1 -> VHAL_OTAProgressRate_enum/1
  LeftShift/1 -> BitwiseOR/1
  UnitConverter1/1 -> LeftShift/1
  Byte_0/1 -> UnitConverter1/1

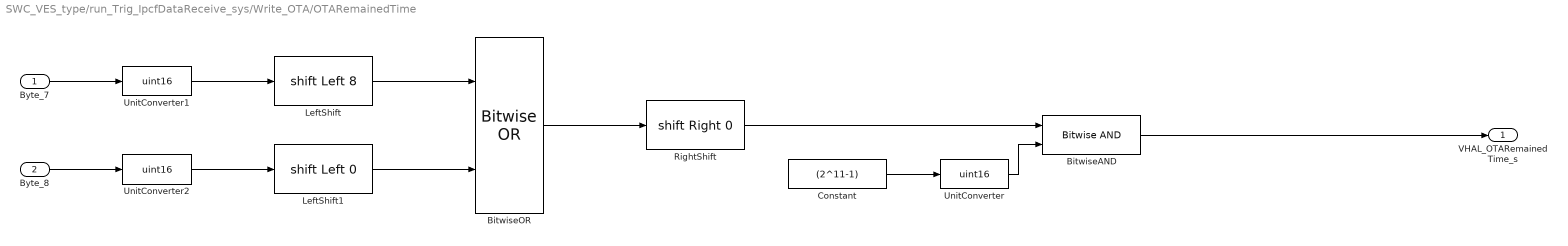
== system SWC_VES_type/run_Trig_IpcfDataReceive_sys/Write_OTA/OTARemainedTime ==
  Byte_7 : Inport
  Byte_8 : Inport  Port=2
  BitwiseAND : simulink/Logic and Bit Operations/Bitwise Operator  logicop=AND  UseBitMask=off  NumInputPorts=2  BitMask=bin2dec('11011001')  BitMaskRealWorld=Stored Integer
  BitwiseOR : simulink/Logic and Bit Operations/Bitwise Operator  logicop=OR  UseBitMask=off  NumInputPorts=2  BitMask=bin2dec('11011001')  BitMaskRealWorld=Stored Integer
  Constant : Constant  Value=(2^11-1)
  LeftShift : ArithShift  BitShiftNumber=8  BitShiftDirection=Left
  LeftShift1 : ArithShift  BitShiftDirection=Left
  RightShift : ArithShift  BitShiftDirection=Right
  UnitConverter : DataTypeConversion  OutDataTypeStr=uint16
  UnitConverter1 : DataTypeConversion  OutDataTypeStr=uint16
  UnitConverter2 : DataTypeConversion  OutDataTypeStr=uint16
  VHAL_OTARemainedTime_s : Outport
  wires:
  Byte_8/1 -> UnitConverter2/1
  UnitConverter2/1 -> LeftShift1/1
  LeftShift1/1 -> BitwiseOR/2
  Byte_7/1 -> UnitConverter1/1
  UnitConverter1/1 -> LeftShift/1
  LeftShift/1 -> BitwiseOR/1
  BitwiseAND/1 -> VHAL_OTARemainedTime_s/1
  Constant/1 -> UnitConverter/1
  UnitConverter/1 -> BitwiseAND/2
  RightShift/1 -> BitwiseAND/1
  BitwiseOR/1 -> RightShift/1

== system SWC_VES_type/run_Trig_IpcfDataReceive_sys/Write_OTA/OTAUpBackcount ==
  Byte_6 : Inport
  BitwiseAND : simulink/Logic and Bit Operations/Bitwise Operator  logicop=AND  UseBitMask=off  NumInputPorts=2  BitMask=bin2dec('11011001')  BitMaskRealWorld=Stored Integer
  BitwiseOR : simulink/Logic and Bit Operations/Bitwise Operator  logicop=OR  UseBitMask=off  BitMask=bin2dec('11011001')  BitMaskRealWorld=Stored Integer
  Constant : Constant  Value=(2^8-1)
  LeftShift : ArithShift  BitShiftDirection=Left
  RightShift : ArithShift  BitShiftDirection=Right
  UnitConverter : DataTypeConversion  OutDataTypeStr=uint8
  UnitConverter1 : DataTypeConversion  OutDataTypeStr=uint8
  VHAL_OTAUpBackcount_enum : Outport
  wires:
  BitwiseOR/1 -> RightShift/1
  RightShift/1 -> BitwiseAND/1
  UnitConverter/1 -> BitwiseAND/2
  Constant/1 -> UnitConverter/1
  BitwiseAND/1 -> VHAL_OTAUpBackcount_enum/1
  LeftShift/1 -> BitwiseOR/1
  UnitConverter1/1 -> LeftShift/1
  Byte_6/1 -> UnitConverter1/1

== system SWC_VES_type/run_Trig_IpcfDataReceive_sys/Write_OTA/OTAUpdateAvailable ==
  Byte_7 : Inport
  BitwiseAND : simulink/Logic and Bit Operations/Bitwise Operator  logicop=AND  UseBitMask=off  NumInputPorts=2  BitMask=bin2dec('11011001')  BitMaskRealWorld=Stored Integer
  BitwiseOR : simulink/Logic and Bit Operations/Bitwise Operator  logicop=OR  UseBitMask=off  BitMask=bin2dec('11011001')  BitMaskRealWorld=Stored Integer
  Constant : Constant  Value=(2^1-1)
  LeftShift : ArithShift  BitShiftDirection=Left
  RightShift : ArithShift  BitShiftNumber=6  BitShiftDirection=Right
  UnitConverter : DataTypeConversion  OutDataTypeStr=uint8
  UnitConverter1 : DataTypeConversion  OutDataTypeStr=uint8
  VHAL_OTAUpdateAvailable_flg : Outport
  wires:
  BitwiseOR/1 -> RightShift/1
  RightShift/1 -> BitwiseAND/1
  UnitConverter/1 -> BitwiseAND/2
  Constant/1 -> UnitConverter/1
  BitwiseAND/1 -> VHAL_OTAUpdateAvailable_flg/1
  LeftShift/1 -> BitwiseOR/1
  UnitConverter1/1 -> LeftShift/1
  Byte_7/1 -> UnitConverter1/1

== system SWC_VES_type/run_Trig_IpcfDataReceive_sys/Write_OTA/OTAUpdatingECU ==
  Byte_2 : Inport
  BitwiseAND : simulink/Logic and Bit Operations/Bitwise Operator  logicop=AND  UseBitMask=off  NumInputPorts=2  BitMask=bin2dec('11011001')  BitMaskRealWorld=Stored Integer
  BitwiseOR : simulink/Logic and Bit Operations/Bitwise Operator  logicop=OR  UseBitMask=off  BitMask=bin2dec('11011001')  BitMaskRealWorld=Stored Integer
  Constant : Constant  Value=(2^8-1)
  LeftShift : ArithShift  BitShiftDirection=Left
  RightShift : ArithShift  BitShiftDirection=Right
  UnitConverter : DataTypeConversion  OutDataTypeStr=uint8
  UnitConverter1 : DataTypeConversion  OutDataTypeStr=uint8
  VHAL_OTAUpdatingECU_enum : Outport
  wires:
  BitwiseOR/1 -> RightShift/1
  RightShift/1 -> BitwiseAND/1
  UnitConverter/1 -> BitwiseAND/2
  Constant/1 -> UnitConverter/1
  BitwiseAND/1 -> VHAL_OTAUpdatingECU_enum/1
  LeftShift/1 -> BitwiseOR/1
  UnitConverter1/1 -> LeftShift/1
  Byte_2/1 -> UnitConverter1/1

== system SWC_VES_type/run_Trig_IpcfDataReceive_sys/Write_OTA/OTA_TBOXResetReq ==
  Byte_3 : Inport
  BitwiseAND : simulink/Logic and Bit Operations/Bitwise Operator  logicop=AND  UseBitMask=off  NumInputPorts=2  BitMask=bin2dec('11011001')  BitMaskRealWorld=Stored Integer
  BitwiseOR : simulink/Logic and Bit Operations/Bitwise Operator  logicop=OR  UseBitMask=off  BitMask=bin2dec('11011001')  BitMaskRealWorld=Stored Integer
  Constant : Constant  Value=(2^1-1)
  LeftShift : ArithShift  BitShiftDirection=Left
  RightShift : ArithShift  BitShiftNumber=6  BitShiftDirection=Right
  UnitConverter : DataTypeConversion  OutDataTypeStr=uint8
  UnitConverter1 : DataTypeConversion  OutDataTypeStr=uint8
  VHAL_OTALockReq_flg : Outport
  wires:
  Byte_3/1 -> UnitConverter1/1
  UnitConverter1/1 -> LeftShift/1
  LeftShift/1 -> BitwiseOR/1
  BitwiseAND/1 -> VHAL_OTALockReq_flg/1
  Constant/1 -> UnitConverter/1
  UnitConverter/1 -> BitwiseAND/2
  RightShift/1 -> BitwiseAND/1
  BitwiseOR/1 -> RightShift/1

== system SWC_VES_type/run_Trig_IpcfDataReceive_sys/Write_TBOX1/AntitheftZero ==
  Byte_2 : Inport
  BitwiseAND : simulink/Logic and Bit Operations/Bitwise Operator  logicop=AND  UseBitMask=off  NumInputPorts=2  BitMask=bin2dec('11011001')  BitMaskRealWorld=Stored Integer
  BitwiseOR : simulink/Logic and Bit Operations/Bitwise Operator  logicop=OR  UseBitMask=off  BitMask=bin2dec('11011001')  BitMaskRealWorld=Stored Integer
  Constant : Constant  Value=(2^4-1)
  LeftShift : ArithShift  BitShiftDirection=Left
  RightShift : ArithShift  BitShiftNumber=4  BitShiftDirection=Right
  UnitConverter : DataTypeConversion  OutDataTypeStr=uint8
  UnitConverter1 : DataTypeConversion  OutDataTypeStr=uint8
  VHAL_AntitheftZero_enum : Outport
  wires:
  BitwiseOR/1 -> RightShift/1
  RightShift/1 -> BitwiseAND/1
  UnitConverter/1 -> BitwiseAND/2
  Constant/1 -> UnitConverter/1
  BitwiseAND/1 -> VHAL_AntitheftZero_enum/1
  LeftShift/1 -> BitwiseOR/1
  UnitConverter1/1 -> LeftShift/1
  Byte_2/1 -> UnitConverter1/1

== system SWC_VES_type/run_Trig_IpcfDataReceive_sys/Write_TBOX1/CbnPreACEnaReq ==
  Byte_5 : Inport
  BitwiseAND : simulink/Logic and Bit Operations/Bitwise Operator  logicop=AND  UseBitMask=off  NumInputPorts=2  BitMask=bin2dec('11011001')  BitMaskRealWorld=Stored Integer
  BitwiseOR : simulink/Logic and Bit Operations/Bitwise Operator  logicop=OR  UseBitMask=off  BitMask=bin2dec('11011001')  BitMaskRealWorld=Stored Integer
  Constant : Constant  Value=(2^2-1)
  LeftShift : ArithShift  BitShiftDirection=Left
  RightShift : ArithShift  BitShiftNumber=6  BitShiftDirection=Right
  UnitConverter : DataTypeConversion  OutDataTypeStr=uint8
  UnitConverter1 : DataTypeConversion  OutDataTypeStr=uint8
  VHAL_CbnPreACEnaReq_enum : Outport
  wires:
  BitwiseOR/1 -> RightShift/1
  RightShift/1 -> BitwiseAND/1
  UnitConverter/1 -> BitwiseAND/2
  Constant/1 -> UnitConverter/1
  BitwiseAND/1 -> VHAL_CbnPreACEnaReq_enum/1
  LeftShift/1 -> BitwiseOR/1
  UnitConverter1/1 -> LeftShift/1
  Byte_5/1 -> UnitConverter1/1

== system SWC_VES_type/run_Trig_IpcfDataReceive_sys/Write_TBOX1/CbnPreReq ==
  Byte_5 : Inport
  BitwiseAND : simulink/Logic and Bit Operations/Bitwise Operator  logicop=AND  UseBitMask=off  NumInputPorts=2  BitMask=bin2dec('11011001')  BitMaskRealWorld=Stored Integer
  BitwiseOR : simulink/Logic and Bit Operations/Bitwise Operator  logicop=OR  UseBitMask=off  BitMask=bin2dec('11011001')  BitMaskRealWorld=Stored Integer
  Constant : Constant  Value=(2^2-1)
  LeftShift : ArithShift  BitShiftDirection=Left
  RightShift : ArithShift  BitShiftNumber=4  BitShiftDirection=Right
  UnitConverter : DataTypeConversion  OutDataTypeStr=uint8
  UnitConverter1 : DataTypeConversion  OutDataTypeStr=uint8
  VHAL_CbnPreReq_enum : Outport
  wires:
  BitwiseOR/1 -> RightShift/1
  RightShift/1 -> BitwiseAND/1
  UnitConverter/1 -> BitwiseAND/2
  Constant/1 -> UnitConverter/1
  BitwiseAND/1 -> VHAL_CbnPreReq_enum/1
  LeftShift/1 -> BitwiseOR/1
  UnitConverter1/1 -> LeftShift/1
  Byte_5/1 -> UnitConverter1/1

== system SWC_VES_type/run_Trig_IpcfDataReceive_sys/Write_TBOX1/CbnPreTarT ==
  Byte_4 : Inport
  BitwiseAND : simulink/Logic and Bit Operations/Bitwise Operator  logicop=AND  UseBitMask=off  NumInputPorts=2  BitMask=bin2dec('11011001')  BitMaskRealWorld=Stored Integer
  BitwiseOR : simulink/Logic and Bit Operations/Bitwise Operator  logicop=OR  UseBitMask=off  BitMask=bin2dec('11011001')  BitMaskRealWorld=Stored Integer
  Constant : Constant  Value=(2^6-1)
  LeftShift : ArithShift  BitShiftDirection=Left
  RightShift : ArithShift  BitShiftDirection=Right
  UnitConverter : DataTypeConversion  OutDataTypeStr=uint8
  UnitConverter1 : DataTypeConversion  OutDataTypeStr=uint8
  VHAL_CbnPreTarT_cnt : Outport
  wires:
  BitwiseOR/1 -> RightShift/1
  RightShift/1 -> BitwiseAND/1
  UnitConverter/1 -> BitwiseAND/2
  Constant/1 -> UnitConverter/1
  BitwiseAND/1 -> VHAL_CbnPreTarT_cnt/1
  LeftShift/1 -> BitwiseOR/1
  UnitConverter1/1 -> LeftShift/1
  Byte_4/1 -> UnitConverter1/1

== system SWC_VES_type/run_Trig_IpcfDataReceive_sys/Write_TBOX1/DrvWdwCtrlCmd ==
  Byte_4 : Inport
  BitwiseAND : simulink/Logic and Bit Operations/Bitwise Operator  logicop=AND  UseBitMask=off  NumInputPorts=2  BitMask=bin2dec('11011001')  BitMaskRealWorld=Stored Integer
  BitwiseOR : simulink/Logic and Bit Operations/Bitwise Operator  logicop=OR  UseBitMask=off  BitMask=bin2dec('11011001')  BitMaskRealWorld=Stored Integer
  Constant : Constant  Value=(2^2-1)
  LeftShift : ArithShift  BitShiftDirection=Left
  RightShift : ArithShift  BitShiftNumber=6  BitShiftDirection=Right
  UnitConverter : DataTypeConversion  OutDataTypeStr=uint8
  UnitConverter1 : DataTypeConversion  OutDataTypeStr=uint8
  VHAL_DrvWdwCtrlCmd_enum : Outport
  wires:
  BitwiseOR/1 -> RightShift/1
  RightShift/1 -> BitwiseAND/1
  UnitConverter/1 -> BitwiseAND/2
  Constant/1 -> UnitConverter/1
  BitwiseAND/1 -> VHAL_DrvWdwCtrlCmd_enum/1
  LeftShift/1 -> BitwiseOR/1
  UnitConverter1/1 -> LeftShift/1
  Byte_4/1 -> UnitConverter1/1

== system SWC_VES_type/run_Trig_IpcfDataReceive_sys/Write_TBOX1/PasWdwCtrlCmd ==
  Byte_8 : Inport
  BitwiseAND : simulink/Logic and Bit Operations/Bitwise Operator  logicop=AND  UseBitMask=off  NumInputPorts=2  BitMask=bin2dec('11011001')  BitMaskRealWorld=Stored Integer
  BitwiseOR : simulink/Logic and Bit Operations/Bitwise Operator  logicop=OR  UseBitMask=off  BitMask=bin2dec('11011001')  BitMaskRealWorld=Stored Integer
  Constant : Constant  Value=(2^7-1)
  LeftShift : ArithShift  BitShiftDirection=Left
  RightShift : ArithShift  BitShiftDirection=Right
  UnitConverter : DataTypeConversion  OutDataTypeStr=uint8
  UnitConverter1 : DataTypeConversion  OutDataTypeStr=uint8
  VHAL_PasWdwCtrlCmd_cnt : Outport
  wires:
  BitwiseOR/1 -> RightShift/1
  RightShift/1 -> BitwiseAND/1
  UnitConverter/1 -> BitwiseAND/2
  Constant/1 -> UnitConverter/1
  BitwiseAND/1 -> VHAL_PasWdwCtrlCmd_cnt/1
  LeftShift/1 -> BitwiseOR/1
  UnitConverter1/1 -> LeftShift/1
  Byte_8/1 -> UnitConverter1/1

== system SWC_VES_type/run_Trig_IpcfDataReceive_sys/Write_TBOX1/PowerOffTSet ==
  Byte_6 : Inport
  BitwiseAND : simulink/Logic and Bit Operations/Bitwise Operator  logicop=AND  UseBitMask=off  NumInputPorts=2  BitMask=bin2dec('11011001')  BitMaskRealWorld=Stored Integer
  BitwiseOR : simulink/Logic and Bit Operations/Bitwise Operator  logicop=OR  UseBitMask=off  BitMask=bin2dec('11011001')  BitMaskRealWorld=Stored Integer
  Constant : Constant  Value=(2^7-1)
  LeftShift : ArithShift  BitShiftDirection=Left
  RightShift : ArithShift  BitShiftDirection=Right
  UnitConverter : DataTypeConversion  OutDataTypeStr=uint8
  UnitConverter1 : DataTypeConversion  OutDataTypeStr=uint8
  VHAL_PowerOffTSet_cnt : Outport
  wires:
  BitwiseOR/1 -> RightShift/1
  RightShift/1 -> BitwiseAND/1
  UnitConverter/1 -> BitwiseAND/2
  Constant/1 -> UnitConverter/1
  BitwiseAND/1 -> VHAL_PowerOffTSet_cnt/1
  LeftShift/1 -> BitwiseOR/1
  UnitConverter1/1 -> LeftShift/1
  Byte_6/1 -> UnitConverter1/1

== system SWC_VES_type/run_Trig_IpcfDataReceive_sys/Write_TBOX1/PowerOffTSet4 ==
  Byte_11 : Inport
  BitwiseAND : simulink/Logic and Bit Operations/Bitwise Operator  logicop=AND  UseBitMask=off  NumInputPorts=2  BitMask=bin2dec('11011001')  BitMaskRealWorld=Stored Integer
  BitwiseOR : simulink/Logic and Bit Operations/Bitwise Operator  logicop=OR  UseBitMask=off  BitMask=bin2dec('11011001')  BitMaskRealWorld=Stored Integer
  Constant : Constant  Value=(2^7-1)
  LeftShift : ArithShift  BitShiftDirection=Left
  RightShift : ArithShift  BitShiftDirection=Right
  UnitConverter : DataTypeConversion  OutDataTypeStr=uint8
  UnitConverter1 : DataTypeConversion  OutDataTypeStr=uint8
  VHAL_PowerOffTSet_cnt : Outport
  wires:
  Byte_11/1 -> UnitConverter1/1
  UnitConverter1/1 -> LeftShift/1
  LeftShift/1 -> BitwiseOR/1
  BitwiseAND/1 -> VHAL_PowerOffTSet_cnt/1
  Constant/1 -> UnitConverter/1
  UnitConverter/1 -> BitwiseAND/2
  RightShift/1 -> BitwiseAND/1
  BitwiseOR/1 -> RightShift/1
